simulink model "haya_cvt_acc"  (R2020a)
settings: Solver=VariableStepAuto  StartTime=0.0  StopTime=100  RelTol=1e-3  EnableMultiTasking=on
libraries: fl_lib x19, sdl_lib x9, nesl_utility x8, simulink x1
settings Model: Creator=kishan  LastModifiedBy=kishan
settings DataIOCC: LimitDataPoints=on  MaxDataPoints=10000
settings OptimizationCC: LifeSpan=inf
settings DebuggingCC: AllowSymbolicDim=off  SFUnexpectedBacktrackingDiag=warning  SFNoUnconditionalDefaultTransitionDiag=warning  SFExecutionAtInitializationDiag=none  ArithmeticOperatorsInVariantConditions=warning
settings SFSimCC: SimUseLocalCustomCode=off  CustomCodeUndefinedFunction=UseInterfaceOnly
settings RTWCC: RTWUseLocalCustomCode=off
settings CodeAppCC: StateflowObjectComments=on
settings GRTTargetCC: TargetLangStandard=C89/C90 (ANSI)
settings ConfigComp: CovMetricSettings=dw  CovHtmlReporting=on  CovSaveCumulativeToWorkspaceVar=on  CovSaveSingleToWorkspaceVar=on  CovExternalEMLEnable=off  CovSFcnEnable=off
settings SimscapeCC: SimscapeLogType=all  SimscapeLogSimulationStatistics=on  SimscapeLogDataHistory=10000

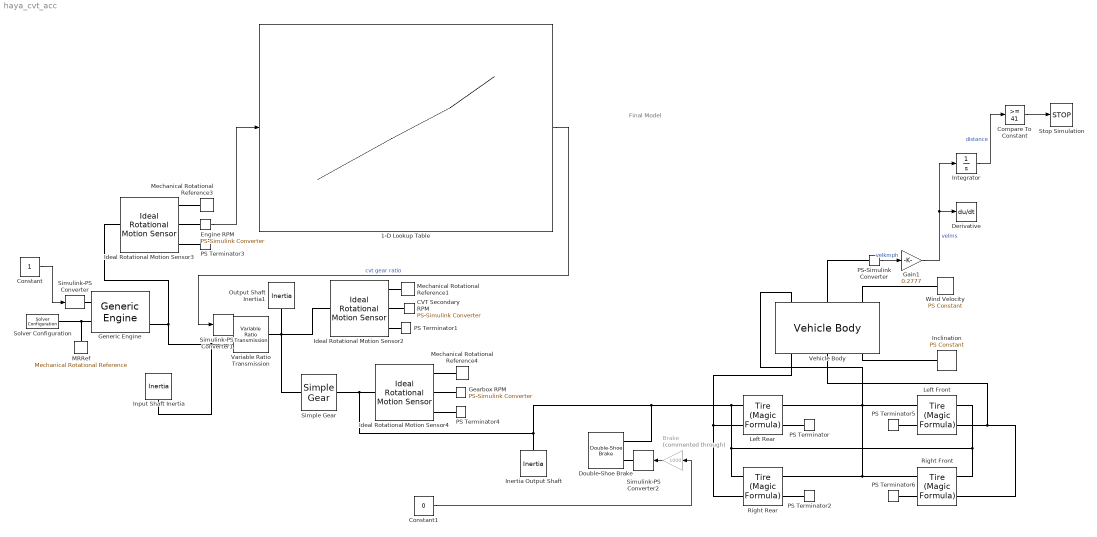
== system haya_cvt_acc ==
  note: Final Model
  1-D Lookup Table : Lookup_n-D  NumberOfTableDimensions=1  BreakpointsForDimension1=[1200,1300,1400,1500,1600,1700,1800,2000,2200,2400,2600,2800,3000,3200,3300,3400,3600,3800,4000]  Table=[3.9,3.9,3.9,3.9,3.9,3.9,3.9,3.9,3.9,3.9,3.9,3.9,3.9,3.9,3.9,3.6,1.3,0.9,0.9]  InternalRulePriority=Speed  RndMeth=Simplest  InputSameDT=on
  Brake : Gain  Commented=through  Gain=1000
  CVT Secondary RPM : nesl_utility/PS-Simulink Converter  PhysicalDomain=network_engine_domain  SubClassName=ps_output  LeftPortType=input  RightPortType=output  PseudoPeriodic=off  Frequencies=[]  Unit=rpm  AffineConversion=off
  Compare To Constant : simulink/Logic and Bit Operations/Compare To Constant  relop=>=  const=41  OutDataTypeStr=boolean
  Constant : Constant
  Constant1 : Constant  Value=0
  Derivative : Derivative
  Double-Shoe Brake : sdl_lib/Brakes & Detents/Rotational/Double-Shoe Brake  r_drum=150 mm  r_act=100 mm  r_pin=125 mm  theta_pin=15 deg  theta_0=5 deg  theta_shoe=120 deg  mu_visc=.01 N*m/(rad/s)  thermal_port=simscape.enum.thermaleffects.omit  mu=0.3  temperature_TLU=[280.0, 300.0, 320.0] K  mu_TLU=[0.1, 0.05, 0.03]  thermal_mass=50 kJ/K  w_thr=0.01 rad/s  temperature_specify=off  temperature_priority=High  temperature=300 K  temperature_nominal_specify=off  temperature_nominal_unit=K  temperature_nominal_value=1
      settings: SourceProductBaseCode=LD  InternalSimscapePortConfiguration="{\"Bottom\":[],\"Left\":[{\"id\":\"F\",\"label\":\"F\",\"type\":\"input\"},{\"id\":\"S\",\"label\":\"S\",\"type\":\"foundation.mechanical.rotational.rotational\"}],\"Right\":[],\"Top\":[]}"
  Engine RPM : nesl_utility/PS-Simulink Converter  PhysicalDomain=network_engine_domain  SubClassName=ps_output  LeftPortType=input  RightPortType=output  PseudoPeriodic=off  Frequencies=[]  Unit=rpm  AffineConversion=off
  Gain1 : Gain  Gain=0.2777
  Gearbox RPM : nesl_utility/PS-Simulink Converter  PhysicalDomain=network_engine_domain  SubClassName=ps_output  LeftPortType=input  RightPortType=output  PseudoPeriodic=off  Frequencies=[]  Unit=rpm  AffineConversion=off
  Generic Engine : sdl_lib/Engines/Generic Engine  model_parameterization=2  engine_type=1  P_max=10 HP_DIN  w_P_max=3600 rpm  w_max=3800 rpm  w_min=2000 rpm  w_tab=[1200,1300,1400,1500,1600,1700,1800,1900,2002.18126875636,2019.21958284649,2039.91189682583,2064.25096548641,2086.15805933638,2106.85037331572,2129.97224703633,2151.88175595563,2175.00604474557,2195.69835872491,2221.25945246409,2246.81330099530,2279.67997944357,2322.27697220356,2358.79282040239,2388.00549896146,2419.65015233113,2454.94639052067,2485.37626401970,2515.80372244940,2549.88518076832,2583.96663908723,2621.69726715670,2663.08431018470,2703.24932813409,2744.63395609277,2790.88977888062,2840.79235634970,2877.31061961786,2911.39207793677,2952.77912096477,2990.51699424222,3022.16406268121,3064.76830064917,3101.28656391733,3143.89563202395,3188.93425987183,3223.02054832940,3264.41242149605,3304.58468465342,3347.19133769071,3392.23238060792,3437.27825366378,3478.66771176111,3511.53922034804,3546.84270374556,3571.19384775276,3595.54257669063,3700,3800] rpm  trq_tab=[17.4223,17.472712,17.654823,17.83694,18.033329,18.21453,18.262472,18.32032,18.3276065237906,18.3620514500430,18.3615382478114,18.4306696072487,18.4649937800348,18.4644805778031,18.5336421256070,18.5330987350088,18.5673927194283,18.5668795171967,18.5662455614988,18.6702142959538,18.6345316466722,18.7032101806110,18.7023045296140,18.7015800088164,18.7356626746700,18.7696547754239,18.7689000662597,18.8030129204798,18.8021676462160,18.8013223719521,18.8352540959728,18.7993601281253,18.8332314754129,18.8322050709496,18.8961903496358,19,18.8940469756096,18.7932017013457,18.7573077334982,18.6866367673660,18.6858518698353,18.6499277136211,18.6141544992398,18.5084952162571,18.4725106833098,18.4019302822774,18.2963011876612,18.2255698447959,18.1547781251975,18.0839260288659,17.9433388057657,17.8725772745338,17.7671594984836,17.6965489090846,17.5913424516004,17.5210035575004,17.284409,17.066967] N*m  pwr_tab=[5.25, 5.75, 6.3, 7, 7.5, 8, 8.4, 8.6, 9] kW  interp_method=simscape.enum.interpolation.linear  model_inertia=1  inertia=0.15 kg*m^2  initial_velocity=1800 rpm  model_time_constant=0  time_constant=0.01 ms  T0=0  w_thr=1 rpm  idle_speed=1  idle_speed_reference=1800 rpm  tau_controller=1 s  idle_w_thr=1 rpm  redline=1  redline_speed=3600 rpm  tau_redline=1 s  redline_w_thr=1 rpm  fc_model=0  fc_per_rev=25 mg/rev  displaced_volume=400 cm^3  rev_per_cycle=2  fc_w_tab=[1000, 2000, 3000, 4000, 5000, 6000] rpm  fc_trq_tab=[0, 80, 160, 200, 240, 320, 360, 400] N*m  fc_tab=[.5, .9, 1.4, 1.6, 1.9, 2.7, 3.4, 4.4; 1, 1.7, 2.7, 3.1, 3.6, 5, 6, 7.4; 1.4, 2.7, 4, 4.8, 5.6, 7.5, 8.5, 10.5; 2, 3.6, 5.8, 6.7, 8, 10.4, 11.7, 13.3; 2.5, 4.8, 7.9, 9.4, 10.8, 14, 16.2, 18.6; 3.1, 6, 10.3, 11.9, 13.8, 18.4, 22, 26.5] g/s  bmep_tab=[0, 250, 500, 625, 750, 1000, 1150, 1250] kPa  bsfc_tab=[410, 380, 300, 280, 270, 290, 320, 380; 410, 370, 290, 270, 260, 270, 285, 320; 415, 380, 290, 275, 265, 270, 270, 300; 420, 390, 310, 290, 285, 280, 280, 285; 430, 410, 340, 320, 310, 300, 310, 320; 450, 430, 370, 340, 330, 330, 350, 380] g/hr/kW  fc_interp_method=simscape.enum.interpolation.linear
      settings: SourceProductBaseCode=LD  LogSimulationData=on  InternalSimscapePortConfiguration="{\"Bottom\":[],\"Left\":[{\"id\":\"T\",\"label\":\"T\",\"type\":\"input\"},{\"id\":\"B\",\"label\":\"B\",\"type\":\"foundation.mechanical.rotational.rotational\"}],\"Right\":[{\"id\":\"P\",\"label\":\"P\",\"type\":\"output\"},{\"id\":\"FC\",\"label\":\"FC\",\"type\":\"output\"},{\"id\":\"F\",\"label\":\"F\",\"type\":\"foundation.mechanical.rotational.rotational\"}],\"Top\":[]}"
  Ideal Rotational Motion Sensor2 : fl_lib/Mechanical/Mechanical Sensors/Ideal Rotational Motion Sensor  wrap_angle=simscape.enum.onoff.off  offset=0 rad
  Ideal Rotational Motion Sensor3 : fl_lib/Mechanical/Mechanical Sensors/Ideal Rotational Motion Sensor  wrap_angle=simscape.enum.onoff.off  offset=0 rad
  Ideal Rotational Motion Sensor4 : fl_lib/Mechanical/Mechanical Sensors/Ideal Rotational Motion Sensor  wrap_angle=simscape.enum.onoff.off  offset=0 rad
  Inclination : fl_lib/Physical Signals/Sources/PS Constant  constant=0
  Inertia Output Shaft : fl_lib/Mechanical/Rotational Elements/Inertia  inertia=0.0001125 kg*m^2  w_specify=on  w_priority=High  w=0 rpm  w_nominal_specify=off  w_nominal_unit=rad/s  w_nominal_value=1  t_specify=off  t_priority=High  t=0 N*m  t_nominal_specify=off  t_nominal_unit=N*m  t_nominal_value=1
  Input Shaft Inertia : fl_lib/Mechanical/Rotational Elements/Inertia  inertia=0.00253 kg*m^2  w_specify=on  w_priority=None  w=2500 rpm  w_nominal_specify=off  w_nominal_unit=rad/s  w_nominal_value=1  t_specify=off  t_priority=High  t=0 N*m  t_nominal_specify=off  t_nominal_unit=N*m  t_nominal_value=1
  Integrator : Integrator
  Left Front : sdl_lib/Tires & Vehicles/Tire (Magic Formula)  parameterization=sdl.enum.magic_tire_model.constant  F_z1=3000 N  F_x1=3500 N  kappa1=10  B_m=5  C_m=1  D_m=0.3  E_m=1  fz0=4000 N  p_Cx=1.685  p_Dx=[1.21, -.037]  p_Ex=[.344, .095, -.02, 0]  p_Kx=[21.51, -.163, .245]  p_Hx=[-.002, .002]  p_Vx=[0, 0]  v_tr_thr=0.1 m/s  r_e=0.292 m  model_compliance=0  stiffness=1e6 N/m  damping=1000 N/(m/s)  model_inertia=1  inertia=0.0667255 kg*m^2  initial_velocity=0 rpm  model_resistance=1  resistance_model=1  coeff=0.02  p_tire=250e3 Pa  alpha=-0.003  beta=0.97  coeff_a=84e-4  coeff_b=6.2e-4 s/m  coeff_c=1.6e-4 s^2/m^2  v_thr=0.001 m/s
  Left Rear : sdl_lib/Tires & Vehicles/Tire (Magic Formula)  parameterization=sdl.enum.magic_tire_model.constant  F_z1=3000 N  F_x1=3500 N  kappa1=10  B_m=5  C_m=0.9  D_m=1  E_m=0.97  fz0=4000 N  p_Cx=1.685  p_Dx=[1.21, -.037]  p_Ex=[.344, .095, -.02, 0]  p_Kx=[21.51, -.163, .245]  p_Hx=[-.002, .002]  p_Vx=[0, 0]  v_tr_thr=0.1 m/s  r_e=0.292 m  model_compliance=0  stiffness=1e6 N/m  damping=1000 N/(m/s)  model_inertia=1  inertia=0.0667255 kg*m^2  initial_velocity=0 rpm  model_resistance=1  resistance_model=1  coeff=0.02  p_tire=250e3 Pa  alpha=-0.003  beta=0.97  coeff_a=84e-4  coeff_b=6.2e-4 s/m  coeff_c=1.6e-4 s^2/m^2  v_thr=0.001 m/s
  MRRef : fl_lib/Mechanical/Rotational Elements/Mechanical Rotational Reference
  Mechanical Rotational Reference1 : fl_lib/Mechanical/Rotational Elements/Mechanical Rotational Reference
  Mechanical Rotational Reference3 : fl_lib/Mechanical/Rotational Elements/Mechanical Rotational Reference
  Mechanical Rotational Reference4 : fl_lib/Mechanical/Rotational Elements/Mechanical Rotational Reference
  Output Shaft Inertia1 : fl_lib/Mechanical/Rotational Elements/Inertia  inertia=0.00243 kg*m^2  w_specify=on  w_priority=None  w=2500 rpm  w_nominal_specify=off  w_nominal_unit=rad/s  w_nominal_value=1  t_specify=off  t_priority=High  t=0 N*m  t_nominal_specify=off  t_nominal_unit=N*m  t_nominal_value=1
  PS Terminator{,1..6} (7 alike) : fl_lib/Physical Signals/Sinks/PS Terminator
  PS-Simulink Converter : nesl_utility/PS-Simulink Converter  PhysicalDomain=network_engine_domain  SubClassName=ps_output  LeftPortType=input  RightPortType=output  PseudoPeriodic=off  Frequencies=[]  Unit=km/hr  AffineConversion=off
  Right Front : sdl_lib/Tires & Vehicles/Tire (Magic Formula)  parameterization=sdl.enum.magic_tire_model.constant  F_z1=3000 N  F_x1=3500 N  kappa1=10  B_m=5  C_m=1  D_m=0.3  E_m=1  fz0=4000 N  p_Cx=1.685  p_Dx=[1.21, -.037]  p_Ex=[.344, .095, -.02, 0]  p_Kx=[21.51, -.163, .245]  p_Hx=[-.002, .002]  p_Vx=[0, 0]  v_tr_thr=0.1 m/s  r_e=0.292 m  model_compliance=0  stiffness=1e6 N/m  damping=1000 N/(m/s)  model_inertia=1  inertia=0.0667255 kg*m^2  initial_velocity=0 rpm  model_resistance=1  resistance_model=1  coeff=0.02  p_tire=250e3 Pa  alpha=-0.003  beta=0.97  coeff_a=84e-4  coeff_b=6.2e-4 s/m  coeff_c=1.6e-4 s^2/m^2  v_thr=0.001 m/s
  Right Rear : sdl_lib/Tires & Vehicles/Tire (Magic Formula)  parameterization=sdl.enum.magic_tire_model.constant  F_z1=3000 N  F_x1=3500 N  kappa1=10  B_m=5  C_m=1  D_m=0.3  E_m=1  fz0=4000 N  p_Cx=1.685  p_Dx=[1.21, -.037]  p_Ex=[.344, .095, -.02, 0]  p_Kx=[21.51, -.163, .245]  p_Hx=[-.002, .002]  p_Vx=[0, 0]  v_tr_thr=0.1 m/s  r_e=0.292 m  model_compliance=0  stiffness=1e6 N/m  damping=1000 N/(m/s)  model_inertia=1  inertia=0.0667255 kg*m^2  initial_velocity=0 rpm  model_resistance=1  resistance_model=1  coeff=0.02  p_tire=250e3 Pa  alpha=-0.003  beta=0.97  coeff_a=84e-4  coeff_b=6.2e-4 s/m  coeff_c=1.6e-4 s^2/m^2  v_thr=0.001 m/s
  Simple Gear : sdl_lib/Gears/Simple Gear  ratio=7.3  rotation_direction=1  friction_model=sdl.enum.gear_efficiencies_load.off  T_noload=0.1 N*m  T_nom=5 N*m  efficiency_nom=0.8  efficiency=0.9  mu_visc=[0, 0] N*m/(rad/s)  w_thr=0.01 rad/s  pwr_thr=0.001 W  enable_faults=simscape.enum.onoff.off  efficiency_fault=0.05  external_fault=simscape.enum.onoff.off  temporal_fault=simscape.enum.onoff.off  fault_time=5 s  fault_angles=pi / 12 rad  report_fault=1  temperature_TLU=[280, 300, 320] K  load_TLU=[1, 5, 10] N*m  efficiency_TLU=[.95, .9, .85]  efficiency_TLU2=[.85, .8, .75; .95, .9, .85; .85, .8, .7]  thermal_mass=50 J/K  T_init=300 K
  Simulink-PS Converter : nesl_utility/Simulink-PS Converter  PhysicalDomain=network_engine_domain  SubClassName=ps_input  LeftPortType=input  RightPortType=output  PseudoPeriodic=off  Frequencies=[]  NoiseDistribution=none  NoiseParameters=[]  Unit=1  AffineConversion=off  FilteringAndDerivatives=zero  SimscapeFilterOrder=1  InputFilterTimeConstant=0.001  UdotUserProvided=1
  Simulink-PS Converter1 : nesl_utility/Simulink-PS Converter  PhysicalDomain=network_engine_domain  SubClassName=ps_input  LeftPortType=input  RightPortType=output  PseudoPeriodic=off  Frequencies=[]  NoiseDistribution=none  NoiseParameters=[]  Unit=1  AffineConversion=off  FilteringAndDerivatives=zero  SimscapeFilterOrder=1  InputFilterTimeConstant=.001  UdotUserProvided=0
  Simulink-PS Converter2 : nesl_utility/Simulink-PS Converter  PhysicalDomain=network_engine_domain  SubClassName=ps_input  LeftPortType=input  RightPortType=output  PseudoPeriodic=off  Frequencies=[]  NoiseDistribution=none  NoiseParameters=[]  Unit=N  AffineConversion=off  FilteringAndDerivatives=zero  SimscapeFilterOrder=1  InputFilterTimeConstant=0.001  UdotUserProvided=1
  Solver Configuration : nesl_utility/Solver Configuration  PhysicalDomain=network_engine_domain  SubClassName=solver  LeftPortType=input  RightPortType=generic  Tones=[]  Harmonics=[]  SimulateNoise=off  Profile=off  UseLocalSampling=off  EnableSwitchedLinearOptims=on  FrequencyDomain=off  UseCCode=off  RelTol=0.001  AbsTol=1e-06  MinStep=1e-09  ToWorkspace=off  RevertToSquareIcSolve=off  NumHomotopyIterations=100  PhasorMode=off  PhasorModeNumHarmonics=1  DoDC=off  ResidualTolerance=1e-9  UseLocalSolver=off  LocalSolverChoice=NE_BACKWARD_EULER_ADVANCER  LocalSolverSampleTime=0.001  DoFixedCost=off  MaxNonlinIter=3  MaxModeIter=2  LinearAlgebra=Sparse  EquationFormulation=NE_TIME_EF  DelaysMemoryBudget=1024  AutomaticFiltering=on  FilteringTimeConstant=0.001  PartitionStorageMethod=AS_NEEDED  PartitionMemoryBudget=1024  PartitionMethod=FAST
  Stop Simulation : Stop
  Variable Ratio Transmission : sdl_lib/Couplings & Drives/Variable Ratio Transmission  rotation_direction=1  kp=3e5 N*m/rad  kv=0.05 N*m/(rad/s)  initial_torque=0 N*m  losses_model=1  efficiency=0.8  mu_visc=[0, 0] N*m/(rad/s)  w_thr=0.01 rad/s  R_specify=off  R_priority=None  R=1  R_nominal_specify=off  R_nominal_unit=1  R_nominal_value=1
      settings: SourceProductBaseCode=LD  InternalSimscapePortConfiguration="{\"Bottom\":[],\"Left\":[{\"id\":\"ratio\",\"label\":\"r\",\"type\":\"input\"},{\"id\":\"B\",\"label\":\"B\",\"type\":\"foundation.mechanical.rotational.rotational\"}],\"Right\":[{\"id\":\"F\",\"label\":\"F\",\"type\":\"foundation.mechanical.rotational.rotational\"}],\"Top\":[]}"
  Vehicle Body : sdl_lib/Tires & Vehicles/Vehicle Body  mass=237 kg  n_w=2  x_f=770.98 mm  x_r=639.02 mm  y_c=491.9 mm  mass_var=simscape.enum.onoff.off  model_pitch=simscape.enum.onoff.off  inertia=4000 kg*m^2  suspension_model=sdl.enum.linearTLU.linear  k_f=1e4 N/m  b_f=1e4 N/(m/s)  k_r=1e4 N/m  b_r=1e4 N/(m/s)  k_f_TLU=[-2000, -1000, 0, 1000, 2000] N  x_f_TLU=[-.4, -.2, 0, .2, .4] m  b_f_TLU=[-200, -100, 0, 100, 200] N  v_f_TLU=[-4, -2, 0, 2, 4] m/s  k_r_TLU=[-2000, -1000, 0, 1000, 2000] N  x_r_TLU=[-.4, -.2, 0, .2, .4] m  b_r_TLU=[-200, -100, 0, 100, 200] N  v_r_TLU=[-4, -2, 0, 2, 4] m/s  interp_method=simscape.enum.interpolation.linear  extrap_method=simscape.enum.extrapolation.linear  model_hardstop=simscape.enum.onoff.off  upper_bound_f=.25 m  lower_bound_f=-.25 m  stop_k_f=1e6 N/m  stop_b_f=150 N/(m/s)  upper_bound_r=.25 m  lower_bound_r=-.25 m  stop_k_r=1e6 N/m  stop_b_r=150 N/(m/s)  initial_pitch=0 rad  initial_pitch_rate=0 rad/s  g=9.81 m/s^2  liftoff_warning=simscape.enum.onoff.off  area=1 m^2  Cd=1.05  rho=1.18 kg/m^3  v_specify=off  v_priority=High  v=0 m/s  v_nominal_specify=off  v_nominal_unit=m/s  v_nominal_value=1
      settings: LogSimulationData=on
  Wind Velocity : fl_lib/Physical Signals/Sources/PS Constant  constant=0
  wires:
  Engine RPM/1 -> 1-D Lookup Table/1
  Constant/1 -> Simulink-PS Converter/1
  Brake/1 -> Simulink-PS Converter2/1
  1-D Lookup Table/1 -> Simulink-PS Converter1/1  "cvt gear ratio"
  PS-Simulink Converter/1 -> Gain1/1  "velkmph"
  Constant1/1 -> Brake/1
  Compare To Constant/1 -> Stop Simulation/1
  Integrator/1 -> Compare To Constant/1  "distance"
  Gain1/1 -> Derivative/1, Integrator/1  "velms"
  connections:
  Ideal Rotational Motion Sensor4/LConn1 -- Simple Gear/RConn1 -- Inertia Output Shaft/LConn1 -- Double-Shoe Brake/LConn2 -- Right Front/LConn2 -- Left Front/LConn2 -- Right Rear/LConn2 -- Left Rear/LConn2
  Input Shaft Inertia/LConn1 -- Generic Engine/RConn3 -- Ideal Rotational Motion Sensor3/LConn1 -- Variable Ratio Transmission/LConn2
  Generic Engine/LConn2 -- Solver Configuration/RConn1 -- MRRef/LConn1
  Right Front/RConn2 -- Left Front/RConn2 -- Left Rear/RConn2 -- Vehicle Body/LConn1 -- Right Rear/RConn2
  Vehicle Body/RConn1 -- Left Rear/LConn1 -- Right Rear/LConn1
  Vehicle Body/RConn2 -- Left Front/LConn1 -- Right Front/LConn1
  Variable Ratio Transmission/RConn1 -- Output Shaft Inertia1/LConn1 -- Simple Gear/LConn1 -- Ideal Rotational Motion Sensor2/LConn1
  Mechanical Rotational Reference1/LConn1 -- Ideal Rotational Motion Sensor2/RConn1
  PS Terminator3/LConn1 -- Ideal Rotational Motion Sensor3/RConn3
  PS Terminator1/LConn1 -- Ideal Rotational Motion Sensor2/RConn3
  Engine RPM/LConn1 -- Ideal Rotational Motion Sensor3/RConn2
  Inclination/RConn1 -- Vehicle Body/RConn3
  CVT Secondary RPM/LConn1 -- Ideal Rotational Motion Sensor2/RConn2
  PS Terminator2/LConn1 -- Right Rear/RConn1
  PS Terminator6/LConn1 -- Right Front/RConn1
  PS-Simulink Converter/LConn1 -- Vehicle Body/LConn2
  Simulink-PS Converter/RConn1 -- Generic Engine/LConn1
  Double-Shoe Brake/LConn1 -- Simulink-PS Converter2/RConn1
  Simulink-PS Converter1/RConn1 -- Variable Ratio Transmission/LConn1
  PS Terminator5/LConn1 -- Left Front/RConn1
  PS Terminator/LConn1 -- Left Rear/RConn1
  Mechanical Rotational Reference4/LConn1 -- Ideal Rotational Motion Sensor4/RConn1
  Mechanical Rotational Reference3/LConn1 -- Ideal Rotational Motion Sensor3/RConn1
  Gearbox RPM/LConn1 -- Ideal Rotational Motion Sensor4/RConn2
  Wind Velocity/RConn1 -- Vehicle Body/LConn3
  PS Terminator4/LConn1 -- Ideal Rotational Motion Sensor4/RConn3
